simulink model "comparator_SARLogic"  (R2018b)
settings: Solver=VariableStepAuto  StartTime=0.0  StopTime=10.0  RelTol=1e-3
libraries: simulink x1
settings Model: Creator=iamcy  LastModifiedBy=iamcy

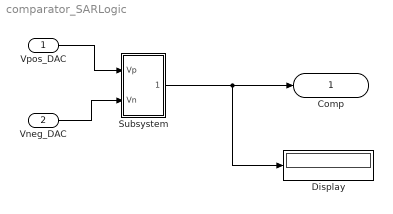
== system comparator_SARLogic ==
  Vpos_DAC : Inport
  Vneg_DAC : Inport  Port=2
  Display : Display
  Subsystem : Subsystem
  Comp : Outport  SignalName=Comp
  wires:
  Vneg_DAC/1 -> Subsystem/2(Vn)
  Subsystem/1(Comp) -> Comp/1, Display/1
  Vpos_DAC/1 -> Subsystem/1(Vp)

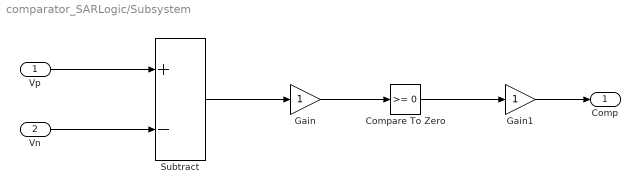
== system comparator_SARLogic/Subsystem ==
  Vp : Inport
  Vn : Inport  Port=2
  Compare To Zero : simulink/Logic and Bit Operations/Compare To Zero  relop=>=  OutDataTypeStr=boolean
  Gain : Gain
  Gain1 : Gain
  Subtract : Sum  Inputs=+-
  Comp : Outport
  wires:
  Gain1/1 -> Comp/1
  Subtract/1 -> Gain/1
  Gain/1 -> Compare To Zero/1
  Compare To Zero/1 -> Gain1/1
  Vn/1 -> Subtract/2
  Vp/1 -> Subtract/1
